simulink model "ConfiguredVirtualVehicleModel"  (R2023b)
settings: configuration reference "VehicleVariable" (kept outside this file)
StartFcn:
  | %tic
StopFcn:
  | %toc
model workspace (MAT data in the model file):
  ExtDrvCmdsSwitch : Simulink.Parameter (value not decoded)
  ExtDrvRefSwitch : Simulink.Parameter (value not decoded)
  ExtEnvSwitch : Simulink.Parameter (value not decoded)
  ExtGndSwitch : Simulink.Parameter (value not decoded)
values from neighbouring files (symbols this model uses):
  L = 2.79    [EVFmincon_custom.m]
symbols that are objects in the model workspace (value not decoded): ExtDrvCmdsSwitch, ExtDrvRefSwitch, ExtEnvSwitch, ExtGndSwitch
undefined symbols (not defined in the file or in its folder): AccelCmd, AmbTemp, BaroPress, CtrlTcuInitGear, CtrlVcuCltch1InitCmd, CurvGradRef, CurvRef, DCM, DecelCmd, Disabled, DriverAeroRes, DriverDrivelineRes, DriverInitialGear, DriverPreviewDist, DriverRollRes, DriverShiftTime, DriverTimeConst, DriverTractiveForce, EnvAbsPrs, EnvAirTemp, EnvGrvty, EnvNomFrictionScaling, EnvNominalGrade, EnvWindVelX, EnvWindVelY, EnvWindVelZ, FTP75, Gnd, Grade, HazzardCmd, HighBeamCmd, lambda_mux, LeftSignalCmd, LngRef, LowBeamCmd, LtrRef, PhiRef, PlntVehDstCGFrntAxl, PlntVehDstCGRearAxl, PlntVehInitLatPos, PlntVehInitLongPos, PlntVehInitPitchAng, PlntVehInitRollAng, PlntVehInitVertPos, PlntVehInitYawAng, PlntVehMass, PlntVehTrckWdth, PlntVehYawMomentInertia, PlntWhlLdRadius, RightSignalCmd, ScnCRMaxLatAccel, ScnCRRadius, ScnDLCGateLongPos, ScnDLCLatRef, ScnDLCLatRefOffset, ScnDLCLongRefBpt, ScnDLCLongRefStartPos, ScnDLCVehicleWidth, ScnFHCounterDwellTime, ScnFHInitialDwellTime ... (+22)
libraries: simulink x27, autolibutils x8, vehdynlibscenariocommon x7, vehdynlibviscommon x3, vehdynlibdriver x2, sim3dgroundtruthsensorlib x2, autolibshared x2, vrlib x1, autolibsharedcommon x1, sharedtransform x1, sim3dlib x1, sim3dautolib x1
(part 4 of 6)

== system ConfiguredVirtualVehicleModel/Environment/Varying Friction/Varying Friction ==
  In1 : Inport
  In2 : Inport  Port=2
  Cg : Inport  Port=3
  Bus Selector : BusSelector  OutputSignals=FrntAxl.Lft.Disp.X,FrntAxl.Rght.Disp.X,RearAxl.Lft.Disp.X,RearAxl.Rght.Disp.X
  Bus Selector1 : BusSelector  OutputSignals=FrntAxl.Lft.Disp.Y,FrntAxl.Rght.Disp.Y,RearAxl.Lft.Disp.Y,RearAxl.Rght.Disp.Y
  Road Track Friction : Subsystem  mask(Road Track Friction){surface_popup=Split friction coefficient scaling factor, lambda_g=EnvNomFrictionScaling, lambda_r=.6, r_x0=175, r_y0=-100, r_xw=1000, r_yw=500, aMode=2}
      mask prompts: surface_popup "Type of surface:"; lambda_g "Scaling factor for the friction coefficient of ground, lambda_g :"; lambda_r "Scaling factor for the friction coefficient of rectangular surface, lambda_r :"; r_x0 "X coordinate of lower left corner of rectangular surface, r_x0 [m]:"; r_y0 "Y coordinate of lower left corner of rectangular surface, r_y0 [m]:"; r_xw "Rectangular surface width in X direction, r_xw [m]:"; r_yw "Rectangular surface width in Y direction, r_yw [m]:"
      mask init:
      | % Scaling factor for the friction coefficient around the rectangular region
      | mutable = [lambda_g, lambda_g, lambda_g, lambda_g;
      |            lambda_g, lambda_r, lambda_r, lambda_g; 
      |            lambda_g, lambda_r, lambda_r, lambda_g; 
      |            lambda_g, lambda_g, lambda_g, lambda_g ];
      |        
      | 
      | % The step is distance between breakpoint near the boundary of high and
      | % low friction coefficient
      | 
      | step = 0.01 ; 
      | 
      | % In the mask initialization, xbr and ybr breakpoints are with respect to
      | % Body fixed coordinate system. At time t=0, xbr and ybr breakpoints
      | % updates to Earth (Inertial) Fixed coordinate system. The breakpoints for
      | % the lookup table are added via inputs.
      | 
      | xbr = [(r_x0 - step) , (r_x0 + step), (r_x0 + r_xw - step) , (r_x0 + r_xw + step) ];
      | ybr = [(r_y0 - step) , (r_y0 + step), (r_y0 + r_yw - step) , (r_y0 + r_yw + step) ];
      | 
      | 
      | % To check if the created track is split mu or constant mu
      | 
      | surface_popup = get_param(gcb, 'surface_popup');
      | 
      | if strcmp(surface_popup, 'Split friction coefficient scaling factor')
      |     SplitLambdaTrck = 1;
      | elseif strcmp(surface_popup, 'Constant friction coefficient scaling factor')
      |     SplitLambdaTrck = 0;
      | end
      mask Help: eval('vdynblkshelp(''vdynblkstrack'')');
      mask TypeOptions surface_popup: Constant friction coefficient scaling factor | Split friction coefficient scaling factor
      mask Callback surface_popup:
      | surface_popup = get_param(gcb, 'surface_popup');
      | m = Simulink.Mask.get(gcb);
      | 
      | lambda_g = m.getParameter('lambda_g');
      | lambda_r = m.getParameter('lambda_r');
      | r_x0 = m.getParameter('r_x0');
      | r_y0 = m.getParameter('r_y0');
      | r_xw = m.getParameter('r_xw');
      | r_yw = m.getParameter('r_yw');
      | %track_view = m.getParameter('track_view');
      | 
      | 
      | if strcmp(surface_popup, 'Split friction coefficient scaling factor')
      |     lambda_g.Visible = 'on';
      |     lambda_r.Visible = 'on';
      |     r_x0.Visible = 'on';
      |     r_y0.Visible = 'on';
      |     r_xw.Visible = 'on';
      |     r_yw.Visible = 'on';
      |     %track_view.Visible = 'on';
      | 
      | elseif strcmp(surface_popup,'Constant friction coefficient scaling factor')
      |     lambda_g.Visible = 'on';
      |     lambda_r.Visible = 'off';
      |     r_x0.Visible = 'off';
      |     r_y0.Visible = 'off';
      |     r_xw.Visible = 'off';
      |     r_yw.Visible = 'off';
      |     %track_view.Visible = 'off';
      | end
      | [~]=autosharedicon('autolibutils',gcb,0);
      mask DialogControl DescGroupVar Prompt: Track description  (mask)
      mask DialogControl DescTextVar Prompt: Generates a default or user-specified track which creates a rectangular surface of specified friction coefficient. The location of rectangular surface is relative to the origin of Body Fixed Coordinate System.The input of the block is X and Y coordinates of the wheel from the vehicle feedback bus. The block output is friction coefficient for all the wheels.
  Wheel Coordinates : Subsystem
  FricCoeffLambda : Outport
  wires:
  Bus Selector1/1 -> Wheel Coordinates/5(FrntAxlLftY)  "<Y>"
  Bus Selector/3 -> Wheel Coordinates/3(RearAxlLftX)  "<X>"
  Bus Selector/4 -> Wheel Coordinates/4(RearAxlRghtX)  "<X>"
  Wheel Coordinates/1(XWhl) -> Road Track Friction/1(XWhl)
  Bus Selector1/2 -> Wheel Coordinates/6(FrntAxlRghtY)  "<Y>"
  Bus Selector/2 -> Wheel Coordinates/2(FrntAxlRghtX)  "<X>"
  Bus Selector/1 -> Wheel Coordinates/1(FrntAxlLftX)  "<X>"
  Bus Selector1/3 -> Wheel Coordinates/7(RearAxlLftY)  "<Y>"
  Bus Selector1/4 -> Wheel Coordinates/8(RearAxlRghtY)  "<Y>"
  Cg/1 -> Road Track Friction/3(Cg)
  Wheel Coordinates/2(YWhl) -> Road Track Friction/2(YWhl)
  Road Track Friction/1(FricCoeffLambda) -> FricCoeffLambda/1
  In1/1 -> Bus Selector/1
  In2/1 -> Bus Selector1/1

== system ConfiguredVirtualVehicleModel/Scenarios/Coordinate Systems/ISO 8855 (Z-up) ==
  ExtDrvRefIn : Inport
  ExtDrvCmdIn : Inport  Port=2
  Bus Assignment : BusAssignment  AssignedSignals=LtrRef,YRef,PhiRef,CurvRef,CurvGradRef
  Bus Assignment1 : BusAssignment  AssignedSignals=SteerCmd.SteerCmd
  Bus Selector : BusSelector  OutputSignals=LtrRef,YRef,PhiRef,CurvRef,CurvGradRef
  Bus Selector1 : BusSelector  OutputSignals=SteerCmd.SteerCmd
  Unary Minus{,1..5} (6 alike) : UnaryMinus
  ExtDrvRef : Outport
  ExtDrvCmd : Outport  Port=2
  wires:
  ExtDrvRefIn/1 -> Bus Assignment/1, Bus Selector/1
  ExtDrvCmdIn/1 -> Bus Assignment1/1, Bus Selector1/1
  Unary Minus/1 -> Bus Assignment/2
  Bus Assignment1/1 -> ExtDrvCmd/1
  Bus Assignment/1 -> ExtDrvRef/1
  Bus Selector/1 -> Unary Minus/1  "<LtrRef>"
  Unary Minus2/1 -> Bus Assignment/3
  Unary Minus3/1 -> Bus Assignment/4
  Unary Minus4/1 -> Bus Assignment/5
  Unary Minus5/1 -> Bus Assignment/6
  Bus Selector/2 -> Unary Minus2/1  "<YRef>"
  Bus Selector/3 -> Unary Minus3/1  "<PhiRef>"
  Bus Selector/4 -> Unary Minus4/1  "<CurvRef>"
  Bus Selector/5 -> Unary Minus5/1  "<CurvGradRef>"
  Unary Minus1/1 -> Bus Assignment1/2
  Bus Selector1/1 -> Unary Minus1/1  "<SteerCmd>"

== system ConfiguredVirtualVehicleModel/Scenarios/Coordinate Systems/SAE J670 (Z-down) ==
  ExtDrvRefIn : Inport
  ExtDrvCmdIn : Inport  Port=2
  ExtDrvRef : Outport
  ExtDrvCmd : Outport  Port=2
  wires:
  ExtDrvCmdIn/1 -> ExtDrvCmd/1
  ExtDrvRefIn/1 -> ExtDrvRef/1

== system ConfiguredVirtualVehicleModel/Scenarios/Reference Generator/Reference Generator ==
  "VehFdbk " : Inport
  3D Engine : Subsystem  Variant=on  VariantControlMode=label  LabelModeActiveChoice=Disabled  mask(3D Engine){engine3D=Disabled, SceneDesc=Open surface, dt3D=dt3D, defaultPos=Recommended for scene, X_o=X_o, Y_o=Y_o, Z_o=Z_o, phi_o=phi_o, theta_o=theta_o, psi_o=psi_o}
      mask prompts: engine3D "3D Engine"; SceneDesc "shared_sim3dblks:sim3dblkConfig:SceneDesc"; dt3D "Engine frame rate, dt3D [s]:"; X_o "Initial longitudinal position, X_o [m]:"; Y_o "Initial lateral position, Y_o [m]:"; Z_o "Initial vertical position, Z_o [m]:"; phi_o "Initial roll angle, phi_o [rad]:"; theta_o "Initial pitch angle, theta_o [rad]:"; psi_o "Initial yaw angle, psi_o [rad]:"
      mask help: This subsystem contains the interface blocks which permit the display of the vehicle in the 3D virtual environment. Enable it to view the simulation progress, disable it to inhibit the display.
      mask init:
      | if ~license('test','vehicle_dynamics_blockset')
      |     return;
      | end
      | GrndFdbkPath = [bdroot(gcb) '/Environment/Ground Feedback'];
      | switch get_param(gcb,'engine3D')    
      |     case 'Disabled'
      |         try
      |             set_param(GrndFdbkPath,'LabelModeActiveChoice','0');
      |             set_param([bdroot(gcb) '/Scenarios/Reference Generator/Reference Generator/Reference Generator/Double Lane Change/Double Lane Change'],'use3DCones','off');
      |             set_param([bdroot(gcb) '/Scenarios/Reference Generator/Reference Generator/Reference Generator/Constant Radius/Constant Radius'],'use3DCones','off');                                   
      |         catch
      |             disp('Warning: Ground feedback source subsystem was not found. Ground feedback source remains unchanged.');
      |         end
      |     case 'Enabled'
      |         try
      |             set_param(GrndFdbkPath,'LabelModeActiveChoice','1'); 
      |             set_param([bdroot(gcb) '/Scenarios/Reference Generator/Reference Generator/Reference Generator/Double Lane Change/Double Lane Change'],'use3DCones','on');
      |             set_param([bdroot(gcb) '/Scenarios/Reference Generator/Reference Generator/Reference Generator/Constant Radius/Constant Radius'],'use3DCones','on');
      |         catch
      |             disp('Warning: Ground feedback source subsystem was not found. Ground feedback source remains unchanged.');
      |         end
      |     otherwise
      | end
      settings: AttributesFormatString=|
      | %<SceneDesc>
      | %<engine3D>
      mask Help: eval('vdynblkshelp(''vdynblks3dengine'')');
      mask TypeOptions engine3D: vdynblks:vehdynRefApp3DEng:blkRdBt_engine3D_c2 | vdynblks:vehdynRefApp3DEng:blkRdBt_engine3D_c1
      mask Callback engine3D:
      | sim3denabled=get_param(gcb,'engine3D');
      | set_param(gcb,'OverrideUsingVariant',sim3denabled);
      mask TypeOptions SceneDesc: 3D Engine/Simulation 3D Scene Configuration/SceneDesc
      mask Callback SceneDesc: [~] = vdynblks3Dsceneconfig(gcb);
      mask TypeOptions defaultPos: vdynblks:vehdynRefApp3DEng:blkRdBt_defaultPos_c1 | vdynblks:vehdynRefApp3DEng:blkRdBt_defaultPos_c2
      mask DialogControl engineConfig Prompt: 3D Engine Settings
      mask DialogControl SceneDesc Prompt: Scene name:
      mask DialogControl posSetup Prompt: Initial vehicle position
      mask DialogControl posSetupDesc Prompt: To use these initial vehicle positions, first Apply the initial values and then click Update the model workspaces with the initial values.
      mask DialogControl setModelPos Prompt: Update model workspaces with initial values
      mask DialogControl setModelPos Callback: [~] = vdynblksmdlWSconfig(gcb);
      mask Display: disp('3D Engine')
  Reference Generator : Subsystem  Variant=on  VariantControlMode=label  VariantControl=Variant1  LabelModeActiveChoice=Drive Cycle
  " Ref" : Outport  VectorParamsAs1DForOutWhenUnconnected=off
  Vis : Outport  Port=2  VectorParamsAs1DForOutWhenUnconnected=off
  " Fdbk" : Outport  Port=3  VectorParamsAs1DForOutWhenUnconnected=off
  wires:
  Reference Generator/3(" Fdbk") -> " Fdbk"/1
  Reference Generator/2(" Ref") -> " Ref"/1
  Reference Generator/1(" Vis") -> Vis/1
  "VehFdbk "/1 -> 3D Engine/1(VehFdbk), Reference Generator/1("VehFdbk ")

== system ConfiguredVirtualVehicleModel/Vehicle/Trailer Input/Ground Info Trailer ==
  Env : Inport
  Ground Info 2 AxleTrailer : Subsystem  VariantControl=0
  Ground Info 3 AxleTrailer : Subsystem  VariantControl=1
  Ground : Outport
  Friction : Outport  Port=2

== system ConfiguredVirtualVehicleModel/Visualization/Coordinate Systems/ISO 8855 (Z-up) ==
  VehFdbkIn : Inport
  Bus Assignment : BusAssignment  AssignedSignals=Body.InertFrm.Cg.Disp.Y,Body.InertFrm.Cg.Disp.Z,Body.InertFrm.Cg.Vel.Ydot,Body.InertFrm.Cg.Vel.Zdot,Body.InertFrm.Geom.Disp.Y,Body.InertFrm.Geom.Disp.Z,Body.InertFrm.Cg.Ang.theta,Body.InertFrm.Cg.Ang.psi,Body.BdyFrm.Cg.Vel.ydot,Body.BdyFrm.Cg.Vel.zdot,Body.BdyFrm.Cg.AngVel.q,Body.BdyFrm.Cg.AngVel.r,Body.BdyFrm.Cg.Acc.ay,Body.BdyFrm.Cg.Acc.az,Body.BdyFrm.Cg.Acc.yddot,Body.BdyFrm.Cg.Acc.zddot
  Bus Selector : BusSelector  OutputSignals=Body.InertFrm.Cg.Disp.Y,Body.InertFrm.Cg.Disp.Z,Body.InertFrm.Cg.Vel.Ydot,Body.InertFrm.Cg.Vel.Zdot,Body.InertFrm.Geom.Disp.Y,Body.InertFrm.Geom.Disp.Z,Body.InertFrm.Cg.Ang.theta,Body.InertFrm.Cg.Ang.psi,Body.BdyFrm.Cg.Vel.ydot,Body.BdyFrm.Cg.Vel.zdot,Body.BdyFrm.Cg.AngVel.q,Body.BdyFrm.Cg.AngVel.r,Body.BdyFrm.Cg.Acc.ay,Body.BdyFrm.Cg.Acc.az,Body.BdyFrm.Cg.Acc.yddot,Body.BdyFrm.Cg.Acc.zddot
  Unary Minus{,1..15} (16 alike) : UnaryMinus
  VehFdbk : Outport
  wires:
  VehFdbkIn/1 -> Bus Assignment/1, Bus Selector/1
  Bus Assignment/1 -> VehFdbk/1
  Bus Selector/1 -> Unary Minus/1  "<Y>"
  Bus Selector/2 -> Unary Minus2/1  "<Z>"
  Bus Selector/11 -> Unary Minus10/1  "<q>"
  Bus Selector/12 -> Unary Minus11/1  "<r>"
  Bus Selector/13 -> Unary Minus12/1  "<ay>"
  Bus Selector/14 -> Unary Minus13/1  "<az>"
  Bus Selector/15 -> Unary Minus14/1  "<yddot>"
  Bus Selector/16 -> Unary Minus15/1  "<zddot>"
  Bus Selector/3 -> Unary Minus3/1  "<Ydot>"
  Bus Selector/4 -> Unary Minus4/1  "<Zdot>"
  Bus Selector/5 -> Unary Minus5/1  "<Y>"
  Bus Selector/6 -> Unary Minus1/1  "<Z>"
  Bus Selector/7 -> Unary Minus6/1  "<theta>"
  Bus Selector/8 -> Unary Minus7/1  "<psi>"
  Bus Selector/9 -> Unary Minus8/1  "<ydot>"
  Bus Selector/10 -> Unary Minus9/1  "<zdot>"
  Unary Minus/1 -> Bus Assignment/2
  Unary Minus2/1 -> Bus Assignment/3
  Unary Minus3/1 -> Bus Assignment/4
  Unary Minus4/1 -> Bus Assignment/5
  Unary Minus8/1 -> Bus Assignment/10
  Unary Minus9/1 -> Bus Assignment/11
  Unary Minus10/1 -> Bus Assignment/12
  Unary Minus11/1 -> Bus Assignment/13
  Unary Minus12/1 -> Bus Assignment/14
  Unary Minus13/1 -> Bus Assignment/15
  Unary Minus14/1 -> Bus Assignment/16
  Unary Minus15/1 -> Bus Assignment/17
  Unary Minus5/1 -> Bus Assignment/6
  Unary Minus1/1 -> Bus Assignment/7
  Unary Minus6/1 -> Bus Assignment/8
  Unary Minus7/1 -> Bus Assignment/9

== system ConfiguredVirtualVehicleModel/Visualization/Coordinate Systems/SAE J670 (Z-down) ==
  VehFdbkIn : Inport
  VehFdbk : Outport
  wires:
  VehFdbkIn/1 -> VehFdbk/1

== system ConfiguredVirtualVehicleModel/Visualization/ISO 15037-1:2006/Disabled ==
  VehFdbk : Inport
  Terminator1 : Terminator
  wires:
  VehFdbk/1 -> Terminator1/1

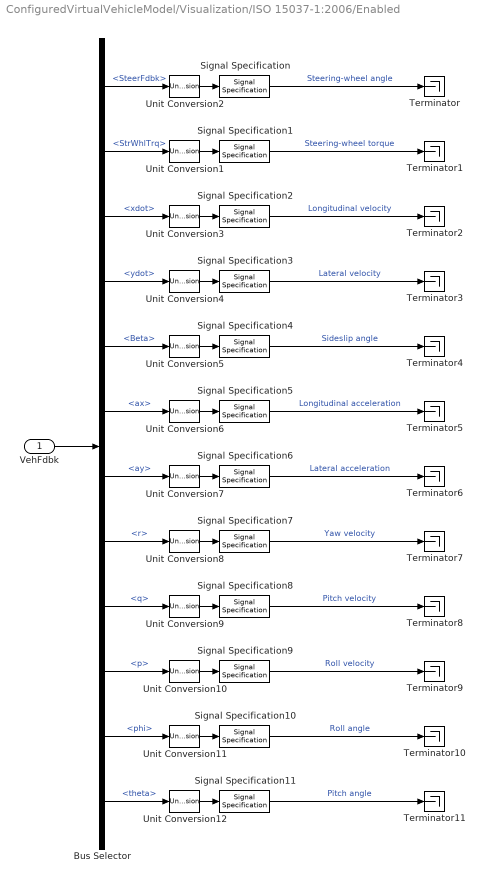
== system ConfiguredVirtualVehicleModel/Visualization/ISO 15037-1:2006/Enabled ==
  VehFdbk : Inport
  Bus Selector : BusSelector  OutputSignals=Driver.SteerFdbk,Steering.StrWhlTrq,Body.BdyFrm.Cg.Vel.xdot,Body.BdyFrm.Cg.Vel.ydot,Body.BdyFrm.Cg.Ang.Beta,Body.BdyFrm.Cg.Acc.ax,Body.BdyFrm.Cg.Acc.ay,Body.BdyFrm.Cg.AngVel.r,Body.BdyFrm.Cg.AngVel.q,Body.BdyFrm.Cg.AngVel.p,Body.InertFrm.Cg.Ang.phi,Body.InertFrm.Cg.Ang.theta
  Signal Specification{,4,10..11} (4 alike) : SignalSpecification  Unit=deg
  Signal Specification1 : SignalSpecification  Unit=N*m
  Signal Specification2 : SignalSpecification  Unit=km/h
  Signal Specification3 : SignalSpecification  Unit=m/s
  Signal Specification5 : SignalSpecification  Unit=m/s^2
  Signal Specification6 : SignalSpecification  Unit=m/s^2
  Signal Specification7 : SignalSpecification  Unit=deg/s
  Signal Specification8 : SignalSpecification  Unit=deg/s
  Signal Specification9 : SignalSpecification  Unit=deg/s
  Terminator{,1..11} (12 alike) : Terminator
  Unit Conversion{1..12} (12 alike) : UnitConversion
  wires:
  Bus Selector/12 -> Unit Conversion12/1  "<theta>"
  Signal Specification11/1 -> Terminator11/1  "Pitch angle"
  Unit Conversion12/1 -> Signal Specification11/1
  Bus Selector/11 -> Unit Conversion11/1  "<phi>"
  Unit Conversion11/1 -> Signal Specification10/1
  Signal Specification10/1 -> Terminator10/1  "Roll angle"
  Bus Selector/10 -> Unit Conversion10/1  "<p>"
  Signal Specification9/1 -> Terminator9/1  "Roll velocity"
  Unit Conversion10/1 -> Signal Specification9/1
  Bus Selector/9 -> Unit Conversion9/1  "<q>"
  Unit Conversion9/1 -> Signal Specification8/1
  Signal Specification8/1 -> Terminator8/1  "Pitch velocity"
  Bus Selector/8 -> Unit Conversion8/1  "<r>"
  Signal Specification7/1 -> Terminator7/1  "Yaw velocity"
  Unit Conversion8/1 -> Signal Specification7/1
  Bus Selector/7 -> Unit Conversion7/1  "<ay>"
  Unit Conversion7/1 -> Signal Specification6/1
  Signal Specification6/1 -> Terminator6/1  "Lateral acceleration"
  Bus Selector/6 -> Unit Conversion6/1  "<ax>"
  Signal Specification5/1 -> Terminator5/1  "Longitudinal acceleration"
  Unit Conversion6/1 -> Signal Specification5/1
  Bus Selector/5 -> Unit Conversion5/1  "<Beta>"
  Unit Conversion5/1 -> Signal Specification4/1
  Signal Specification4/1 -> Terminator4/1  "Sideslip angle"
  Bus Selector/4 -> Unit Conversion4/1  "<ydot>"
  Signal Specification3/1 -> Terminator3/1  "Lateral velocity"
  Unit Conversion4/1 -> Signal Specification3/1
  Bus Selector/3 -> Unit Conversion3/1  "<xdot>"
  Unit Conversion3/1 -> Signal Specification2/1
  Signal Specification2/1 -> Terminator2/1  "Longitudinal velocity"
  Signal Specification1/1 -> Terminator1/1  "Steering-wheel torque"
  Unit Conversion1/1 -> Signal Specification1/1
  Bus Selector/2 -> Unit Conversion1/1  "<StrWhlTrq>"
  Signal Specification/1 -> Terminator/1  "Steering-wheel angle"
  Unit Conversion2/1 -> Signal Specification/1
  VehFdbk/1 -> Bus Selector/1
  Bus Selector/1 -> Unit Conversion2/1  "<SteerFdbk>"

== system ConfiguredVirtualVehicleModel/Visualization/Scope Type/DLC ==
  VehFdbk : Inport
  Vis : Inport  Port=2
  Bus Creator : BusCreator  Inputs=3
  Bus Selector3 : BusSelector  OutputSignals=Body.InertFrm.Cg.Disp.X,Body.InertFrm.Cg.Disp.Z
  Bus Selector4 : BusSelector  OutputSignals=LeftBnd,RightBnd,LtrlRef
  Lane Change : Scope
  Mux1 : Mux  Inputs=3
  Rate Transition : RateTransition  OutPortSampleTime=.1
  Rate Transition1 : RateTransition  OutPortSampleTime=.1
  Rate Transition3 : RateTransition  OutPortSampleTime=.1
  Signal Copy : SignalConversion  OverrideOpt=off
  Signal Copy1 : SignalConversion  OverrideOpt=off
  Signal Copy2 : SignalConversion  OverrideOpt=off
  Ref : Outport  VectorParamsAs1DForOutWhenUnconnected=off
  wires:
  VehFdbk/1 -> Bus Selector3/1
  Vis/1 -> Bus Selector4/1
  Bus Creator/1 -> Ref/1
  Bus Selector3/2 -> Signal Copy2/1  "<Z>"
  Signal Copy/1 -> Bus Creator/2  "YRef"
  Signal Copy1/1 -> Bus Creator/1  "XRef"
  Signal Copy2/1 -> Bus Creator/3  "ZRef"
  Rate Transition3/1 -> Mux1/2  "Right Boundary"
  Bus Selector4/3 -> Signal Copy/1, Rate Transition1/1  "<LtrlRef>"
  Mux1/1 -> Lane Change/1
  Bus Selector4/1 -> Rate Transition/1  "<LeftBnd>"
  Rate Transition/1 -> Mux1/1  "Left Boundary"
  Bus Selector4/2 -> Rate Transition3/1  "<RightBnd>"
  Bus Selector3/1 -> Signal Copy1/1  "<X>"
  Rate Transition1/1 -> Mux1/3  "Reference"

== system ConfiguredVirtualVehicleModel/Visualization/Scope Type/None ==
  VehFdbk : Inport
  Vis : Inport  Port=2
  Bus Selector2 : BusSelector  OutputSignals=Driver.SteerFdbk
  Bus Selector9 : BusSelector  OutputSignals=Body.BdyFrm.Cg.AngVel.r
  Signal Specification1 : SignalSpecification  Unit=rad/s
  Signal Specification3 : SignalSpecification  Unit=deg/s
  Unit Conversion4 : UnitConversion
  Yaw Rate and Steer : Scope  NumInputPorts=2
  Ref : Outport  VectorParamsAs1DForOutWhenUnconnected=off
  wires:
  Bus Selector9/1 -> Signal Specification1/1  "<r>"
  Signal Specification3/1 -> Yaw Rate and Steer/1
  Unit Conversion4/1 -> Signal Specification3/1
  VehFdbk/1 -> Bus Selector2/1, Bus Selector9/1  "VehFdbk"
  Bus Selector2/1 -> Yaw Rate and Steer/2  "<SteerFdbk>"
  Vis/1 -> Ref/1
  Signal Specification1/1 -> Unit Conversion4/1

== system ConfiguredVirtualVehicleModel/Visualization/Scope Type/XYZ ==
  VehFdbk : Inport
  Vis : Inport  Port=2
  Terminator : Terminator
  Ref : Outport  VectorParamsAs1DForOutWhenUnconnected=off
  wires:
  Vis/1 -> Ref/1
  VehFdbk/1 -> Terminator/1

== system ConfiguredVirtualVehicleModel/Visualization/Vehicle XY Plotter/Disabled ==

== system ConfiguredVirtualVehicleModel/Visualization/Vehicle XY Plotter/XY View ==
  Bus Element In2 : Inport  PortName=VehFdbk
  Bus Selector1 : BusSelector  OutputSignals=Body.InertFrm.Cg.Ang.phi,Body.InertFrm.Cg.Ang.theta,Body.InertFrm.Cg.Ang.psi  OutputAsBus=on
  Bus Selector10 : BusSelector  OutputSignals=Wheels.Wheels.Fx,Wheels.Wheels.Fy
  Bus Selector5 : BusSelector  OutputSignals=Steering.Front.WhlAng.FL,Steering.Front.WhlAng.FR,Steering.Rear.WhlAng.RL,Steering.Rear.WhlAng.RR  OutputAsBus=on
  Bus Selector6 : BusSelector  OutputSignals=Body.InertFrm.Geom.Disp.X,Body.InertFrm.Geom.Disp.Y,Body.InertFrm.Geom.Disp.Z  OutputAsBus=on
  Bus Selector7 : BusSelector  OutputSignals=Body.InertFrm.Geom.Vel.Xdot,Body.InertFrm.Geom.Vel.Ydot,Body.InertFrm.Geom.Vel.Zdot  OutputAsBus=on
  Bus Selector9 : BusSelector  OutputSignals=Driveline.EngSpd,Driveline.TransInfo.TransInfo.Trans.TransGear  OutputAsBus=on
  Bus to Vector{,1..4} (5 alike) : BusToVector
  Vehicle XY Plotter : vehdynlibviscommon/Vehicle XY Plot Configuration  extRef=off  extStats=on  extTireF=on  a=PlntVehDstCGFrntAxl  b=PlntVehDstCGRearAxl  w=PlntVehTrckWdth(1)  figBorder=10  bufferSize=1024  velNorm=5  tireFNorm=1000  pltDT=.1
  wires:
  Bus Selector7/1 -> Bus to Vector1/1
  Bus Selector5/1 -> Bus to Vector4/1
  Bus Selector10/2 -> Vehicle XY Plotter/7  "<Fy>"
  Bus to Vector1/1 -> Vehicle XY Plotter/3
  Bus Selector10/1 -> Vehicle XY Plotter/6  "<Fx>"
  Bus Selector1/1 -> Bus to Vector2/1
  Bus Selector9/1 -> Bus to Vector3/1
  Bus to Vector3/1 -> Vehicle XY Plotter/5
  Bus to Vector/1 -> Vehicle XY Plotter/1
  Bus Selector6/1 -> Bus to Vector/1
  Bus to Vector2/1 -> Vehicle XY Plotter/2
  Bus Element In2/1 -> Bus Selector10/1, Bus Selector9/1, Bus Selector5/1, Bus Selector7/1, Bus Selector1/1, Bus Selector6/1  "VehFdbk"
  Bus to Vector4/1 -> Vehicle XY Plotter/4

== system ConfiguredVirtualVehicleModel/Visualization/Vehicle XY Plotter/XY View Ref ==
  Bus Element In2 : Inport  PortName=VehFdbk
  Bus Element In1 : Inport  Port=2  PortName=Ref  Element=YRef
  Bus Element In3 : Inport  Port=2  PortName=Ref  Element=XRef
  Bus Selector1 : BusSelector  OutputSignals=Body.InertFrm.Cg.Ang.phi,Body.InertFrm.Cg.Ang.theta,Body.InertFrm.Cg.Ang.psi  OutputAsBus=on
  Bus Selector10 : BusSelector  OutputSignals=Wheels.Wheels.Fx,Wheels.Wheels.Fy
  Bus Selector5 : BusSelector  OutputSignals=Steering.Front.WhlAng.FL,Steering.Front.WhlAng.FR,Steering.Rear.WhlAng.RL,Steering.Rear.WhlAng.RR  OutputAsBus=on
  Bus Selector6 : BusSelector  OutputSignals=Body.InertFrm.Geom.Disp.X,Body.InertFrm.Geom.Disp.Y,Body.InertFrm.Geom.Disp.Z  OutputAsBus=on
  Bus Selector7 : BusSelector  OutputSignals=Body.InertFrm.Geom.Vel.Xdot,Body.InertFrm.Geom.Vel.Ydot,Body.InertFrm.Geom.Vel.Zdot  OutputAsBus=on
  Bus Selector9 : BusSelector  OutputSignals=Driveline.EngSpd,Driveline.TransInfo.TransInfo.Trans.TransGear  OutputAsBus=on
  Bus to Vector{,1..3} (4 alike) : BusToVector
  Ground1 : Ground
  Mux : Mux  Inputs=3
  Vehicle XY Plotter : vehdynlibviscommon/Vehicle XY Plot Configuration  extRef=on  extStats=on  extTireF=on  a=PlntVehDstCGFrntAxl  b=PlntVehDstCGRearAxl  w=PlntVehTrckWdth(1)  figBorder=10  bufferSize=1024  velNorm=5  tireFNorm=1000  pltDT=.1
  wires:
  Bus Selector7/1 -> Bus to Vector1/1
  Bus Selector5/1 -> Vehicle XY Plotter/4
  Ground1/1 -> Mux/3
  Bus Selector10/2 -> Vehicle XY Plotter/8  "<Fy>"
  Bus to Vector1/1 -> Vehicle XY Plotter/3
  Bus Selector10/1 -> Vehicle XY Plotter/7  "<Fx>"
  Bus Selector1/1 -> Bus to Vector2/1
  Bus Selector9/1 -> Bus to Vector3/1
  Bus Element In1/1 -> Mux/2
  Bus to Vector3/1 -> Vehicle XY Plotter/6
  Bus Element In3/1 -> Mux/1
  Mux/1 -> Vehicle XY Plotter/5
  Bus to Vector/1 -> Vehicle XY Plotter/1
  Bus Selector6/1 -> Bus to Vector/1
  Bus to Vector2/1 -> Vehicle XY Plotter/2
  Bus Element In2/1 -> Bus Selector10/1, Bus Selector9/1, Bus Selector5/1, Bus Selector7/1, Bus Selector1/1, Bus Selector6/1  "VehFdbk"

== system ConfiguredVirtualVehicleModel/Driver Commands/Driver Commands/Dashboard Widgets/Widget Sinks ==
  VehFdbk : Inport
  Bus Selector : BusSelector  OutputSignals=Driver.LightsFdbk.HighBeamFdbk,Driver.LightsFdbk.LowBeamFdbk,Driver.LightsFdbk.LeftSignalFdbk,Driver.LightsFdbk.RightSignalFdbk,Driver.LightsFdbk.HazzardFdbk
  Terminator{,1..4} (5 alike) : Terminator
  wires:
  VehFdbk/1 -> Bus Selector/1
  Bus Selector/1 -> Terminator/1  "<HighBeamFdbk>"
  Bus Selector/2 -> Terminator1/1  "<LowBeamFdbk>"
  Bus Selector/4 -> Terminator3/1  "<RightSignalFdbk>"
  Bus Selector/3 -> Terminator2/1  "<LeftSignalFdbk>"
  Bus Selector/5 -> Terminator4/1  "<HazzardFdbk>"

== system ConfiguredVirtualVehicleModel/Driver Commands/Driver Commands/Dashboard Widgets/Widget Sources ==
  Accelerator : Constant  Value=0  SampleTime=-1
  Brake : Constant  Value=0  SampleTime=-1
  Bus Assignment : BusAssignment  AssignedSignals=HighBeamCmd,LowBeamCmd,LeftSignalCmd,RightSignalCmd,HazzardCmd
  Bus Creator1 : BusCreator  Inputs=6
  Compare To Constant : simulink/Logic and Bit Operations/Compare To Constant  relop===  const=3  OutDataTypeStr=boolean  ZeroCross=off
  Compare To Constant1 : simulink/Logic and Bit Operations/Compare To Constant  relop===  const=2  OutDataTypeStr=boolean  ZeroCross=off
  Compare To Constant2 : simulink/Logic and Bit Operations/Compare To Constant  relop===  const=-1  OutDataTypeStr=boolean  ZeroCross=off
  Compare To Constant3 : simulink/Logic and Bit Operations/Compare To Constant  relop===  const=1  OutDataTypeStr=boolean  ZeroCross=off
  Data Type Conversion : DataTypeConversion  SaturateOnIntegerOverflow=off  RndMeth=Floor
  Gear : Constant  Value=80  SampleTime=-1
  Hazzard : Constant  Value=0  OutDataTypeStr=boolean
  Headlights : Constant  Value=0
  IgnSwtch : Constant  Value=0
  Scaled Wheel Angle Limit [deg] : Gain  Gain=2*360/90
  Signal Lights : Constant  Value=0
  Signal Specification : SignalSpecification  Unit=1
  Signal Specification1 : SignalSpecification  Unit=1
  Signal Specification2 : SignalSpecification  Unit=1
  Signal Specification3 : SignalSpecification  Unit=deg
  Signal Specification4 : SignalSpecification  OutDataTypeStr=boolean  Unit=1
  Signal Specification5 : SignalSpecification  Unit=rad
  Steer : Constant  Value=0  SampleTime=-1
  To Virtual Bus : SignalConversion  ConversionOutput=Virtual bus  OverrideOpt=off
  Unit Conversion : UnitConversion
  VVCLightsCmd : Constant  Value=0  OutDataTypeStr=Bus: VVCLightsCmd  SampleTime=-1
  Driver : Outport
  wires:
  Compare To Constant1/1 -> Bus Assignment/3
  Signal Specification/1 -> Bus Creator1/2  "AccelCmd"
  Signal Specification1/1 -> Bus Creator1/3  "DecelCmd"
  Steer/1 -> Scaled Wheel Angle Limit [deg]/1
  Headlights/1 -> Compare To Constant1/1, Compare To Constant/1
  IgnSwtch/1 -> Data Type Conversion/1
  Accelerator/1 -> Signal Specification/1
  Unit Conversion/1 -> Signal Specification5/1
  Compare To Constant/1 -> Bus Assignment/2
  VVCLightsCmd/1 -> Bus Assignment/1  "LightsCmd"
  Compare To Constant3/1 -> Bus Assignment/5
  Signal Specification2/1 -> Bus Creator1/4  "GearCmd"
  Signal Lights/1 -> Compare To Constant3/1, Compare To Constant2/1
  Hazzard/1 -> Bus Assignment/6
  Brake/1 -> Signal Specification1/1
  To Virtual Bus/1 -> Bus Creator1/6  "LightsCmd"
  Gear/1 -> Signal Specification2/1
  Signal Specification3/1 -> Unit Conversion/1
  Compare To Constant2/1 -> Bus Assignment/4
  Signal Specification5/1 -> Bus Creator1/1  "SteerCmd"
  Bus Assignment/1 -> To Virtual Bus/1
  Bus Creator1/1 -> Driver/1
  Signal Specification4/1 -> Bus Creator1/5  "IgnSwtch"
  Data Type Conversion/1 -> Signal Specification4/1
  Scaled Wheel Angle Limit [deg]/1 -> Signal Specification3/1

== system ConfiguredVirtualVehicleModel/Driver Commands/Driver Commands/Game Wheel Hardware/Paddle Shift ==
  Buttons : Inport
  Add1 : Sum  Inputs=+-+
  Current Gear : UnitDelay  SampleTime=-1  HasFrameUpgradeWarning=on
  Data Type Conversion2 : DataTypeConversion  OutDataTypeStr=double  SaturateOnIntegerOverflow=off  RndMeth=Floor
  Demux2 : Demux  Outputs=2
  Detect Increase2 : simulink/Logic and Bit Operations/Detect Increase  vinit=0.0  OutDataTypeStr=boolean
  Logical Operator1 : Logic  Operator=XOR  Inputs=1  AllPortsSameDT=off  OutDataTypeStr=boolean
  Min/Max Gear : Saturate  UpperLimit=10  LowerLimit=-1
  Selector : Selector  InputPortWidth=32  IndexOptions=Index vector (dialog)  Indices=[5 6]  OutputSizes=1
  Switch2 : Switch  Criteria=u2 > Threshold  SaturateOnIntegerOverflow=off  InputSameDT=off
  Gear : Outport  VectorParamsAs1DForOutWhenUnconnected=off
  wires:
  Add1/1 -> Min/Max Gear/1
  Current Gear/1 -> Add1/3, Switch2/3
  Switch2/1 -> Gear/1, Current Gear/1  "Gear"
  Demux2/1 -> Add1/1
  Demux2/2 -> Add1/2
  Data Type Conversion2/1 -> Demux2/1
  Detect Increase2/1 -> Data Type Conversion2/1, Logical Operator1/1
  Logical Operator1/1 -> Switch2/2
  Min/Max Gear/1 -> Switch2/1
  Buttons/1 -> Selector/1
  Selector/1 -> Detect Increase2/1

== system ConfiguredVirtualVehicleModel/Driver Commands/Driver Commands/Game Wheel Hardware/Stick Shift ==
  Buttons : Inport
  Gain : Gain  Gain=[-1 1:6]
  Selector1 : Selector  InputPortWidth=32  IndexOptions=Index vector (dialog)  Indices=[12:18]  OutputSizes=1
  Sum : Sum  Inputs=+
  Gear : Outport  VectorParamsAs1DForOutWhenUnconnected=off
  wires:
  Selector1/1 -> Gain/1
  Gain/1 -> Sum/1
  Buttons/1 -> Selector1/1
  Sum/1 -> Gear/1

== system ConfiguredVirtualVehicleModel/Driver Commands/Driver Commands/Longitudinal Driver/Hill Hold & Stop ==
  LngRef : Inport
  <EnblDecelCmd> : Inport  Port=2
  <DecelOvrCmd> : Inport  Port=3
  <DecelHld> : Inport  Port=4
  <DecelZero> : Inport  Port=5
  Env : Inport  Port=6
  VehFdbk : Inport  Port=7
  Bus Selector : BusSelector  OutputSignals=Engine.EngSpdOut,Body.BdyFrm.Cg.Vel.xdot,Battery.BattSoc
  Bus Selector1 : BusSelector  OutputSignals=Body.BdyFrm.Cg.Vel.xdot
  Bus Selector2 : BusSelector  OutputSignals=Grade
  Hill Hold : Subsystem
  Logical Operator4 : Logic  Operator=OR  AllPortsSameDT=off  OutDataTypeStr=boolean
  Max : MinMax  Function=max  Inputs=2  ZeroCross=off
  Stop Detection : Subsystem
  Switch : Switch  Criteria=u2 > Threshold  SaturateOnIntegerOverflow=off  InputSameDT=off
  Switch1 : Switch  Criteria=u2 > Threshold  SaturateOnIntegerOverflow=off  InputSameDT=off
  VehFdbk1 : InportShadow  Port=7
  EnblDecelOvr : Outport
  DecelOvrCmd : Outport  Port=2
  DecelHld : Outport  Port=3
  DecelZero : Outport  Port=4
  VelFdbk : Outport  Port=5
  Grade : Outport  Port=6
  wires:
  <DecelHld>/1 -> DecelHld/1
  <DecelZero>/1 -> DecelZero/1
  VehFdbk1/1 -> Bus Selector1/1
  Bus Selector2/1 -> Grade/1, Hill Hold/5(<Grade>)  "<Grade>"
  Env/1 -> Bus Selector2/1
  <DecelOvrCmd>/1 -> Switch1/1
  VehFdbk/1 -> Bus Selector/1
  LngRef/1 -> Stop Detection/1(LngRef), Hill Hold/4(LngRef)
  Bus Selector1/1 -> Stop Detection/2(<xdot>), VelFdbk/1  "<xdot>"
  Max/1 -> Switch1/3
  <EnblDecelCmd>/1 -> Switch/2, Switch/1, Switch1/2
  Switch/1 -> EnblDecelOvr/1
  Switch1/1 -> DecelOvrCmd/1
  Logical Operator4/1 -> Switch/3
  Stop Detection/2(EnblDecelOvr) -> Logical Operator4/2
  Stop Detection/1(DecelOvrCmd) -> Max/2
  Bus Selector/1 -> Hill Hold/1(<EngSpdOut>)  "<EngSpdOut>"
  Bus Selector/2 -> Hill Hold/2(<xdot>)  "<xdot>"
  Bus Selector/3 -> Hill Hold/3(<BattSoc>)  "<BattSoc>"
  Hill Hold/2(EnblDecelOvr) -> Max/1
  Hill Hold/1(DecelOvr) -> Logical Operator4/1

== system ConfiguredVirtualVehicleModel/Driver Commands/Driver Commands/Longitudinal Driver/Longitudinal Driver ==
  VelRef : Inport  Unit=m/s
  EnblAccelOvr : Inport  Port=2
  AccelOvrCmd : Inport  Port=3
  AccelHld : Inport  Port=4
  AccelZero : Inport  Port=5
  EnblDecelOvr : Inport  Port=6
  DecelOvrCmd : Inport  Port=7
  DecelHld : Inport  Port=8
  DecelZero : Inport  Port=9
  VelFdbk : Inport  Port=10  Unit=m/s
  Grade : Inport  Port=11
  ExtGearGround : Ground
  External Action Routing : Subsystem
  Longitudinal Driver : autolibsharedcommon/Longitudinal Driver  cntrlType=PI  shftType=Reverse, Neutral, Drive  vnom=vnom  Kp=Kp  Ki=Ki  Kaw=Kaw  Kff=Kff  Kg=Kg  tauerr=tauerr  tShift=tShift  tRev=tRev  tPark=tPark  pdlVec=pdlVec  upShftTbl=upShftTbl  dwnShftTbl=dwnShftTbl  GearInit=GearInit  tClutch=tClutch  VehVelVec=VehVelVec  KffVec=KffVec  KiVec=KiVec  KpVec=KpVec  KgVec=KgVec  m=m  Kpt=Kpt  Lvv=L  g=g  UpGearVec=UpGearVec  DownGearVec=DownGearVec  aMode=6  errUnit=m/s  aR=aR  bR=bR  cR=cR  tauPt=tauPt
      settings: LibrarySourceBlock=autolibshared/Longitudinal Driver/Longitudinal Driver
  Info : Outport  InitialOutput=0  VectorParamsAs1DForOutWhenUnconnected=off
  AccelCmd : Outport  Port=2  VectorParamsAs1DForOutWhenUnconnected=off
  DecelCmd : Outport  Port=3  VectorParamsAs1DForOutWhenUnconnected=off
  GearCmd : Outport  Port=4
  wires:
  VelRef/1 -> Longitudinal Driver/1
  VelFdbk/1 -> Longitudinal Driver/2
  Longitudinal Driver/1 -> Info/1
  Longitudinal Driver/2 -> AccelCmd/1
  Longitudinal Driver/3 -> DecelCmd/1
  Grade/1 -> Longitudinal Driver/3
  External Action Routing/1(ExtActions) -> Longitudinal Driver/5
  ExtGearGround/1 -> Longitudinal Driver/4
  Longitudinal Driver/4 -> GearCmd/1
  EnblAccelOvr/1 -> External Action Routing/1(EnblAccelOvr)
  AccelOvrCmd/1 -> External Action Routing/2(AccelOvrCmd)
  AccelHld/1 -> External Action Routing/3(AccelHld)
  AccelZero/1 -> External Action Routing/4(AccelZero)
  EnblDecelOvr/1 -> External Action Routing/5(EnblDecelOvr)
  DecelOvrCmd/1 -> External Action Routing/6(DecelOvrCmd)
  DecelHld/1 -> External Action Routing/7(DecelHld)
  DecelZero/1 -> External Action Routing/8(DecelZero)

== system ConfiguredVirtualVehicleModel/Driver Commands/Driver Commands/Predictive Driver/Hill Hold & Stop ==
  LngRef : Inport
  <EnblDecelCmd> : Inport  Port=2
  <DecelOvrCmd> : Inport  Port=3
  <DecelHld> : Inport  Port=4
  <DecelZero> : Inport  Port=5
  Env : Inport  Port=6
  VehFdbk : Inport  Port=7
  Bus Selector : BusSelector  OutputSignals=Engine.EngSpdOut,Body.BdyFrm.Cg.Vel.xdot,Battery.BattSoc
  Bus Selector1 : BusSelector  OutputSignals=Body.BdyFrm.Cg.Vel.xdot
  Bus Selector2 : BusSelector  OutputSignals=Grade
  Hill Hold : Subsystem
  Logical Operator4 : Logic  Operator=OR  AllPortsSameDT=off  OutDataTypeStr=boolean
  Max : MinMax  Function=max  Inputs=2
  Stop Detection : Subsystem
  Switch : Switch  Criteria=u2 > Threshold  SaturateOnIntegerOverflow=off  InputSameDT=off
  Switch1 : Switch  Criteria=u2 > Threshold  SaturateOnIntegerOverflow=off  InputSameDT=off
  VehFdbk1 : InportShadow  Port=7
  EnblDecelOvr : Outport
  DecelOvrCmd : Outport  Port=2
  DecelHld : Outport  Port=3
  DecelZero : Outport  Port=4
  Grade : Outport  Port=5
  VelFdbk : Outport  Port=6
  wires:
  <DecelHld>/1 -> DecelHld/1
  <DecelZero>/1 -> DecelZero/1
  VehFdbk1/1 -> Bus Selector1/1
  Bus Selector2/1 -> Grade/1, Hill Hold/5(<Grade>)  "<Grade>"
  Env/1 -> Bus Selector2/1
  <DecelOvrCmd>/1 -> Switch1/1
  VehFdbk/1 -> Bus Selector/1
  LngRef/1 -> Stop Detection/1(LngRef), Hill Hold/4(LngRef)
  Bus Selector1/1 -> Stop Detection/2(<xdot>), VelFdbk/1  "<xdot>"
  Max/1 -> Switch1/3
  <EnblDecelCmd>/1 -> Switch/2, Switch/1, Switch1/2
  Switch/1 -> EnblDecelOvr/1
  Switch1/1 -> DecelOvrCmd/1
  Logical Operator4/1 -> Switch/3
  Stop Detection/2(EnblDecelOvr) -> Logical Operator4/2
  Stop Detection/1(DecelOvrCmd) -> Max/2
  Bus Selector/1 -> Hill Hold/1(<EngSpdOut>)  "<EngSpdOut>"
  Bus Selector/2 -> Hill Hold/2(<xdot>)  "<xdot>"
  Bus Selector/3 -> Hill Hold/3(<BattSoc>)  "<BattSoc>"
  Hill Hold/2(EnblDecelOvr) -> Max/1
  Hill Hold/1(DecelOvr) -> Logical Operator4/1

== system ConfiguredVirtualVehicleModel/Driver Commands/Driver Commands/Predictive Stanley Driver/Hill Hold & Stop ==
  LngRef : Inport
  <EnblDecelCmd> : Inport  Port=2
  <DecelOvrCmd> : Inport  Port=3
  <DecelHld> : Inport  Port=4
  <DecelZero> : Inport  Port=5
  <CurvRef> : Inport  Port=6
  Env : Inport  Port=7
  VehFdbk : Inport  Port=8
  Bus Selector : BusSelector  OutputSignals=Engine.EngSpdOut,Body.BdyFrm.Cg.Vel.xdot,Battery.BattSoc
  Bus Selector1 : BusSelector  OutputSignals=Body.BdyFrm.Cg.Vel.xdot
  Bus Selector2 : BusSelector  OutputSignals=Grade
  Hill Hold : Subsystem
  Logical Operator4 : Logic  Operator=OR  AllPortsSameDT=off  OutDataTypeStr=boolean
  Max : MinMax  Function=max  Inputs=2
  Stop Detection : Subsystem
  Switch : Switch  Criteria=u2 > Threshold  SaturateOnIntegerOverflow=off  InputSameDT=off
  Switch1 : Switch  Criteria=u2 > Threshold  SaturateOnIntegerOverflow=off  InputSameDT=off
  VehFdbk1 : InportShadow  Port=8
  EnblDecelOvr : Outport
  DecelOvrCmd : Outport  Port=2
  DecelHld : Outport  Port=3
  DecelZero : Outport  Port=4
  Grade : Outport  Port=5
  CurvRef : Outport  Port=6
  VelFdbk : Outport  Port=7
  wires:
  <DecelHld>/1 -> DecelHld/1
  <DecelZero>/1 -> DecelZero/1
  VehFdbk1/1 -> Bus Selector1/1
  Bus Selector2/1 -> Grade/1, Hill Hold/5(<Grade>)  "<Grade>"
  Env/1 -> Bus Selector2/1
  <DecelOvrCmd>/1 -> Switch1/1
  VehFdbk/1 -> Bus Selector/1
  <CurvRef>/1 -> CurvRef/1
  LngRef/1 -> Stop Detection/1(LngRef), Hill Hold/4(LngRef)
  Bus Selector1/1 -> Stop Detection/2(<xdot>), VelFdbk/1  "<xdot>"
  Max/1 -> Switch1/3
  <EnblDecelCmd>/1 -> Switch/2, Switch/1, Switch1/2
  Switch/1 -> EnblDecelOvr/1
  Switch1/1 -> DecelOvrCmd/1
  Logical Operator4/1 -> Switch/3
  Stop Detection/2(EnblDecelOvr) -> Logical Operator4/2
  Stop Detection/1(DecelOvrCmd) -> Max/2
  Bus Selector/1 -> Hill Hold/1(<EngSpdOut>)  "<EngSpdOut>"
  Bus Selector/2 -> Hill Hold/2(<xdot>)  "<xdot>"
  Bus Selector/3 -> Hill Hold/3(<BattSoc>)  "<BattSoc>"
  Hill Hold/2(EnblDecelOvr) -> Max/1
  Hill Hold/1(DecelOvr) -> Logical Operator4/1

== system ConfiguredVirtualVehicleModel/Environment/Ground Feedback/3D Engine/3D Engine Source ==
  WheelFdbk : Inport
  Multiple Points : Subsystem  VariantControl=terrType==2
  Single Point : Subsystem  VariantControl=terrType ==1
  z : Outport
  DCM : Outport  Port=2

== system ConfiguredVirtualVehicleModel/Environment/Subsystem/Estimated Grade/Variant Subsystem ==
  note: 1) Add Subsystem or Model blocks as valid variant choices.
      | 2) You cannot connect blocks at this level. At simulation, connectivity is automatically
      | determined, based on the active variant and port name matching.
  Gnd : Inport
  Three-Axle : Subsystem  VariantControl=ThreeAxle
  Two-Axle : Subsystem  VariantControl=TwoAxle
  F : Outport
  R : Outport  Port=2

== system ConfiguredVirtualVehicleModel/Environment/Subsystem/Variant Subsystem/Three-Axle ==
  InGnd : Inport
  Bus Selector1 : BusSelector  OutputSignals=z.G_FL_z,z.G_FR_z,z.G_ML_z,z.G_MR_z,z.G_RL_z,z.G_RR_z,DCM,mu.mu_FL,mu.mu_FR,mu.mu_ML,mu.mu_MR,mu.mu_RL,mu.mu_RR
  Mux : Mux  Inputs=6
  Mux1 : Mux  Inputs=6
  z : Outport
  <DCM> : Outport  Port=2
  lambda_mux : Outport  Port=3
  wires:
  Bus Selector1/12 -> Mux1/5  "<mu_RL>"
  Bus Selector1/7 -> <DCM>/1  "<DCM>"
  InGnd/1 -> Bus Selector1/1
  Bus Selector1/10 -> Mux1/3  "<mu_ML>"
  Bus Selector1/4 -> Mux/4  "<G_MR_z>"
  Bus Selector1/5 -> Mux/5  "<G_RL_z>"
  Bus Selector1/3 -> Mux/3  "<G_ML_z>"
  Bus Selector1/2 -> Mux/2  "<G_FR_z>"
  Bus Selector1/9 -> Mux1/2  "<mu_FR>"
  Bus Selector1/6 -> Mux/6  "<G_RR_z>"
  Mux/1 -> z/1
  Bus Selector1/11 -> Mux1/4  "<mu_MR>"
  Bus Selector1/1 -> Mux/1  "<G_FL_z>"
  Bus Selector1/13 -> Mux1/6  "<mu_RR>"
  Mux1/1 -> lambda_mux/1
  Bus Selector1/8 -> Mux1/1  "<mu_FL>"

== system ConfiguredVirtualVehicleModel/Environment/Subsystem/Variant Subsystem/Two-Axle ==
  InGnd : Inport
  Bus Selector1 : BusSelector  OutputSignals=z.G_FL_z,z.G_FR_z,z.G_RL_z,z.G_RR_z,DCM,mu.mu_FL,mu.mu_FR,mu.mu_RL,mu.mu_RR
  Mux : Mux
  Mux1 : Mux
  z : Outport
  <DCM> : Outport  Port=2
  lambda_mux : Outport  Port=3
  wires:
  Bus Selector1/9 -> Mux1/4  "<mu_RR>"
  InGnd/1 -> Bus Selector1/1
  Bus Selector1/8 -> Mux1/3  "<mu_RL>"
  Bus Selector1/1 -> Mux/1  "<G_FL_z>"
  Bus Selector1/3 -> Mux/3  "<G_RL_z>"
  Bus Selector1/7 -> Mux1/2  "<mu_FR>"
  Bus Selector1/2 -> Mux/2  "<G_FR_z>"
  Bus Selector1/6 -> Mux1/1  "<mu_FL>"
  Bus Selector1/4 -> Mux/4  "<G_RR_z>"
  Mux1/1 -> lambda_mux/1
  Mux/1 -> z/1
  Bus Selector1/5 -> <DCM>/1  "<DCM>"

== system ConfiguredVirtualVehicleModel/Environment/Varying Friction/Varying Friction/Road Track Friction ==
  XWhl : Inport
  YWhl : Inport  Port=2
  Cg : Inport  Port=3
  2D Lookup Tbl for Scaling Fctr (Lambda) : Subsystem  TreatAsAtomicUnit=on
      mask init:
      | [~]=vehdynicon('vehdynblk',gcb);
  Bus Selector : BusSelector  OutputSignals=X,Y
  Cnst Lambda : Constant  Value=ones(4,1).*lambda_g
  Constant1 : Constant  Value=SplitLambdaTrck
  Creating Inertial Frm Bpt : Subsystem
  En at t = 0 : Subsystem
  "Lambda (t = 0) " : Memory  InitialCondition=ones(4,1).*lambda_g  InheritSampleTime=on
  Switch : Switch  Criteria=u2 > Threshold  SaturateOnIntegerOverflow=off  InputSameDT=off
  FricCoeffLambda : Outport
  wires:
  YWhl/1 -> 2D Lookup Tbl for Scaling Fctr (Lambda)/2(YWhl)
  XWhl/1 -> 2D Lookup Tbl for Scaling Fctr (Lambda)/1(XWhl)
  2D Lookup Tbl for Scaling Fctr (Lambda)/1(Lambda for each whl) -> Switch/1
  "Lambda (t = 0) "/1 -> FricCoeffLambda/1
  Switch/1 -> "Lambda (t = 0) "/1
  Cnst Lambda/1 -> Switch/3
  Constant1/1 -> Switch/2
  Cg/1 -> Bus Selector/1
  Creating Inertial Frm Bpt/1(XBpt) -> 2D Lookup Tbl for Scaling Fctr (Lambda)/3(XBpt)
  Creating Inertial Frm Bpt/2(YBpt) -> 2D Lookup Tbl for Scaling Fctr (Lambda)/4(YBpt)
  Bus Selector/1 -> Creating Inertial Frm Bpt/1(XCg)  "<X>"
  Bus Selector/2 -> Creating Inertial Frm Bpt/2(YCg)  "<Y>"
  En at t = 0/1(Out1) -> Creating Inertial Frm Bpt/Enable

== system ConfiguredVirtualVehicleModel/Environment/Varying Friction/Varying Friction/Wheel Coordinates ==
  FrntAxlLftX : Inport
  FrntAxlRghtX : Inport  Port=2
  RearAxlLftX : Inport  Port=3
  RearAxlRghtX : Inport  Port=4
  FrntAxlLftY : Inport  Port=5
  FrntAxlRghtY : Inport  Port=6
  RearAxlLftY : Inport  Port=7
  RearAxlRghtY : Inport  Port=8
  Matrix Concatenate : Concatenate  NumInputs=4  Mode=Multidimensional array
  Matrix Concatenate1 : Concatenate  NumInputs=4  Mode=Multidimensional array
  XWhl : Outport
  YWhl : Outport  Port=2
  wires:
  RearAxlRghtX/1 -> Matrix Concatenate/4
  Matrix Concatenate/1 -> XWhl/1
  RearAxlRghtY/1 -> Matrix Concatenate1/4
  RearAxlLftX/1 -> Matrix Concatenate/3
  RearAxlLftY/1 -> Matrix Concatenate1/3
  FrntAxlRghtX/1 -> Matrix Concatenate/2
  FrntAxlRghtY/1 -> Matrix Concatenate1/2
  FrntAxlLftY/1 -> Matrix Concatenate1/1
  FrntAxlLftX/1 -> Matrix Concatenate/1
  Matrix Concatenate1/1 -> YWhl/1

== system ConfiguredVirtualVehicleModel/Scenarios/Reference Generator/Reference Generator/3D Engine ==
  note: 1) Add Subsystem or Model blocks as valid variant choices.
      | 2) You cannot connect blocks at this level. At simulation, connectivity is automatically
      | determined, based on the active variant and port name matching.
  VehFdbk : Inport
  3D Engine : Subsystem  VariantControl=Enabled
  3D Engine Disabled : Subsystem  VariantControl=Disabled

== system ConfiguredVirtualVehicleModel/Scenarios/Reference Generator/Reference Generator/Reference Generator ==
  "VehFdbk " : Inport
  Braking : Subsystem  VariantControl=Braking
  Constant Radius : Subsystem  VariantControl=Constant Radius
  Double Lane Change : Subsystem  VariantControl=Double Lane Change
  Drive Cycle : Subsystem  VariantControl=Drive Cycle
  Fishhook : Subsystem  VariantControl=Fishhook
  Increasing Steer : Subsystem  VariantControl=Increasing Steer
  No Commands : Subsystem  VariantControl=No Commands
  Sine with Dwell : Subsystem  VariantControl=Sine with Dwell
  Swept Sine : Subsystem  VariantControl=Swept Sine
  WOT : Subsystem  VariantControl=WOT
  " Vis" : Outport  VectorParamsAs1DForOutWhenUnconnected=off
  " Ref" : Outport  Port=2  VectorParamsAs1DForOutWhenUnconnected=off
  " Fdbk" : Outport  Port=3  VectorParamsAs1DForOutWhenUnconnected=off

== system ConfiguredVirtualVehicleModel/Vehicle/Trailer Input/Ground Info Trailer/Ground Info 2 AxleTrailer ==
  Env : Inport
  Bus Selector1 : BusSelector  OutputSignals=TraGnd.z.G_FL_z,TraGnd.z.G_FR_z,TraGnd.z.G_RL_z,TraGnd.z.G_RR_z
  Bus Selector3 : BusSelector  OutputSignals=Gnd.mu.mu_FL,Gnd.mu.mu_FR,Gnd.mu.mu_RL,Gnd.mu.mu_RR
  Vector Concatenate : Concatenate  NumInputs=4
  Vector Concatenate1 : Concatenate  NumInputs=4
  Ground : Outport
  Friction : Outport  Port=2
  wires:
  Bus Selector3/4 -> Vector Concatenate/4  "<mu_RR>"
  Bus Selector3/3 -> Vector Concatenate/3  "<mu_RL>"
  Bus Selector1/1 -> Vector Concatenate1/1  "<G_FL_z>"
  Bus Selector1/2 -> Vector Concatenate1/2  "<G_FR_z>"
  Bus Selector1/3 -> Vector Concatenate1/3  "<G_RL_z>"
  Bus Selector1/4 -> Vector Concatenate1/4  "<G_RR_z>"
  Bus Selector3/2 -> Vector Concatenate/2  "<mu_FR>"
  Bus Selector3/1 -> Vector Concatenate/1  "<mu_FL>"
  Vector Concatenate/1 -> Friction/1
  Vector Concatenate1/1 -> Ground/1
  Env/1 -> Bus Selector1/1, Bus Selector3/1

== system ConfiguredVirtualVehicleModel/Vehicle/Trailer Input/Ground Info Trailer/Ground Info 3 AxleTrailer ==
  Env : Inport
  Bus Selector1 : BusSelector  OutputSignals=TraGnd.z.G_FL_z,TraGnd.z.G_FR_z,TraGnd.z.G_RL_z,TraGnd.z.G_RR_z,TraGnd.z.G_RL_z,TraGnd.z.G_RR_z
  Bus Selector3 : BusSelector  OutputSignals=TraGnd.mu.mu_FL,TraGnd.mu.mu_FR,TraGnd.mu.mu_RL,TraGnd.mu.mu_RR,TraGnd.mu.mu_RL,TraGnd.mu.mu_RR
  Vector Concatenate : Concatenate  NumInputs=6
  Vector Concatenate1 : Concatenate  NumInputs=6
  Ground : Outport
  Friction : Outport  Port=2
  wires:
  Env/1 -> Bus Selector3/1, Bus Selector1/1
  Vector Concatenate1/1 -> Ground/1
  Vector Concatenate/1 -> Friction/1
  Bus Selector3/1 -> Vector Concatenate/1  "<mu_FL>"
  Bus Selector3/2 -> Vector Concatenate/2  "<mu_FR>"
  Bus Selector3/3 -> Vector Concatenate/3  "<mu_RL>"
  Bus Selector3/4 -> Vector Concatenate/4  "<mu_RR>"
  Bus Selector3/5 -> Vector Concatenate/5  "<mu_RL>"
  Bus Selector3/6 -> Vector Concatenate/6  "<mu_RR>"
  Bus Selector1/1 -> Vector Concatenate1/1  "<G_FL_z>"
  Bus Selector1/2 -> Vector Concatenate1/2  "<G_FR_z>"
  Bus Selector1/3 -> Vector Concatenate1/3  "<G_RL_z>"
  Bus Selector1/4 -> Vector Concatenate1/4  "<G_RR_z>"
  Bus Selector1/5 -> Vector Concatenate1/5  "<G_RL_z>"
  Bus Selector1/6 -> Vector Concatenate1/6  "<G_RR_z>"
